simulink model "sm_motor_grader"  (R2026a)
settings: Solver=daessc  StopTime=stopTime  FixedStep=0.01  AbsTol=1e-3
PostLoadFcn:
  | warning off SimulinkBlock:Foundation:RuntimeAccessInvalidSource
InitFcn:
  | sm_motor_grader_config_initLinkBarHole([bdroot '/Motor Grader'],motGradParams)
StartFcn:
  | tic
StopFcn:
  | Elapsed_Sim_Time = toc;
undefined symbols (not defined in the file): Art, Center, Circle, FL, FR, Grid, LiftL, LiftR, LnL, LnR, Loads, motGradParams, Pin, RFL, RFR, RRL, RRR, Side, StrL, StrR, Tilt, Wheels
libraries: sm_motor_grader_lib x23, sm_lib x11, nesl_utility x10, fl_lib x2, sm_vehicle_utilities_lib x2
(part 2 of 2)

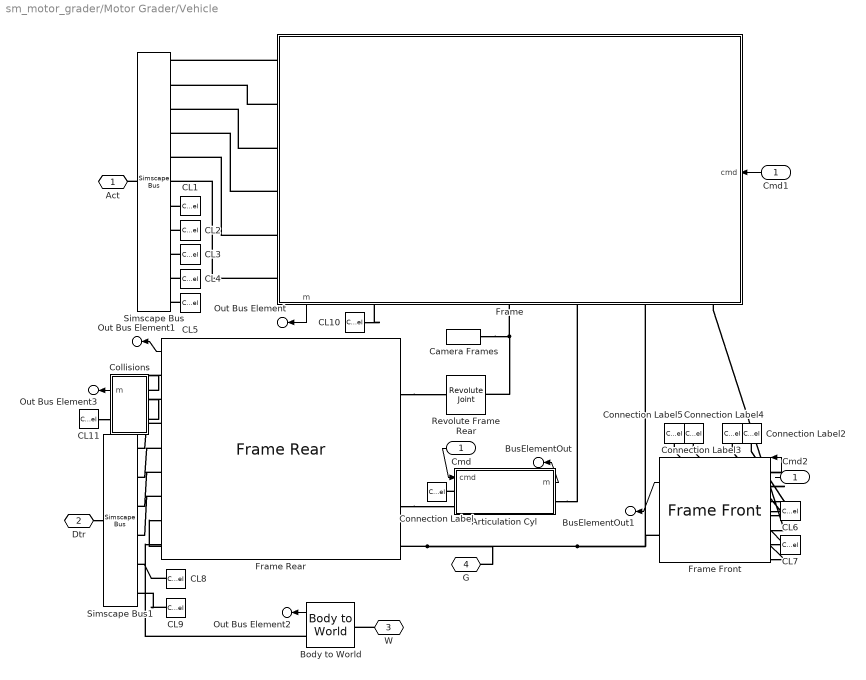
== system sm_motor_grader/Motor Grader/Vehicle ==
  Cmd : Inport
  Articulation Cyl : Subsystem  mask{popup_actuator_model=Position}
      mask prompts: popup_actuator_model "Actuation Mode"
      mask init:
      | bh = gcb;
      | if(strcmp(get_param(bh,'popup_actuator_model'),'Shaft'))
      |     set_param([bh '/Actuator'],'LabelModeActiveChoice','Shaft')
      | else
      |     set_param([bh '/Actuator'],'LabelModeActiveChoice','Position')
      | end
      settings: AttributesFormatString=%<popup_actuator_model>
      mask TypeOptions popup_actuator_model: Position | Shaft
      mask Display:
      | bh = gcb;
      | if(strcmp(get_param(bh,'popup_actuator_model'),'Position'))
      |     image('sm_motor_grader_actuator_intfPosition_IMAGE.png')
      | else
      |     image('sm_motor_grader_actuator_intfShaft_IMAGE.png')
      | end
      | %image('sm_motor_grader_articCylRod_IMAGE.png')
  Body to World : sm_vehicle_utilities_lib/Body to World  Init=Init.Vehicle  SpecifyPosTarget=on
  CL1 : ConnectionLabel  Label=Art
  CL10 : ConnectionLabel  Label=Gbl
  CL11 : ConnectionLabel  Label=Gbl
  CL2 : ConnectionLabel  Label=StrL
  CL3 : ConnectionLabel  Label=LnL
  CL4 : ConnectionLabel  Label=LnR
  CL5 : ConnectionLabel  Label=StrR
  CL6 : ConnectionLabel  Label=FL
  CL7 : ConnectionLabel  Label=FR
  CL8 : ConnectionLabel  Label=FL
  CL9 : ConnectionLabel  Label=FR
  Camera Frames : sm_vehicle_utilities_lib/Camera Frames  Camera=Camera  popup_dolly_camera=Off
  Cmd1 : InportShadow
  Cmd2 : InportShadow
  Collisions : Subsystem
  Connection Label : ConnectionLabel  Label=Art
  Connection Label2 : ConnectionLabel  Label=StrR
  Connection Label3 : ConnectionLabel  Label=LnR
  Connection Label4 : ConnectionLabel  Label=LnL
  Connection Label5 : ConnectionLabel  Label=StrL
  Frame : Subsystem  mask{popup_actuator_model=Position, popup_actuator_model_lift=Position, popup_initial_hole=Center, popup_blade_ground_contact=Loads}
      mask prompts: popup_actuator_model "Actuation Mode"; popup_actuator_model_lift "Actuation Mode Lift"; popup_initial_hole "Link Bar Initial Hole"; popup_blade_ground_contact "Blade Ground Contact"
      mask init:
      | bh = gcb;
      | 
      | modestr = get_param(bh,'popup_actuator_model');
      | set_param([bh '/Blade'],'popup_actuator_model',modestr)
      | set_param([bh '/Drawbar'],'popup_actuator_model',modestr)
      | set_param([bh '/LiftAssembly'],'popup_actuator_model',modestr)
      | 
      | liftmodestr = get_param(bh,'popup_actuator_model_lift');
      | set_param([bh '/LiftAssembly'],'popup_actuator_model_lift',liftmodestr)
      settings: PortSchema="{\"entries\":[{\"content\":{\"sides\":[{\"content\":{},\"type\":\"ConnectorPlacement.EquallySpacedRectSide\",\"uuid\":\"956ff1aa-cf24-496e-9779-d98cb55dab7e\"},{\"content\":{\"connectorIds\":[\"Out1\",\"RConn1\",\"RConn2\",\"RConn3\",\"RConn4\",\"RConn5\",\"RConn6\"],\"side\":\"RIGHT\"},\"type\":\"ConnectorPlacement.EquallySpacedRectSide\",\"uuid\":\"9c9b4268-8eee-41b9-b50a-4033054aa2f0\"},{\"content\":{\"connectorIds\":[\"LConn1\",\"LConn2\",\"LConn3\",\"LConn4\",\"LConn5\",\"LConn6\"],\"side\":\"TOP\"},\"type\":\"ConnectorPlacement.EquallySpacedRectSide\",\"uuid\":\"ed4b7b74-ed0a-49ca-b139-bba335fa3413\"},{\"content\":{\"connectorIds\":[\"In1\"],\"side\":\"BOTTOM\"},\"type\":\"ConnectorPlacement.EquallySpacedRectSide\",\"uuid\":\"cd037d6e-8d6c-4a0e-a629-b4586db15f4a\"}]},\"type\":\"ConnectorPlacement.EquallySpacedConnector\",\"uuid\":\"3490148e-7dca-48b7-9597-0781f6c140f1\"}],\"packageUris\":[\"http://schema.mathworks.com/mf0/Connector/R2020b\"],\"version\":\"1.0\"}"
      mask TypeOptions popup_actuator_model: Position | Shaft
      mask TypeOptions popup_actuator_model_lift: Position | Shaft
      mask TypeOptions popup_initial_hole: LiftAssembly/popup_initial_hole
      mask TypeOptions popup_blade_ground_contact: Blade/popup_blade_ground_contact
      mask Display: image('sm_motor_grader_frameCabBlade_IMAGE.png')
  Frame Front : sm_motor_grader_lib/Frame Front  popup_actuator_model=Position  popup_ground_contact=Magic Formula
  Frame Rear : sm_motor_grader_lib/Frame Rear  popup_ground_contact=Magic Formula
  Revolute Frame Rear : sm_lib/Joints/Revolute Joint  JointMode=Normal  CompositeWrenchDir=FollowerOnBase  CompositeWrenchFrame=BaseFrame  SenseConstraintForce=off  SenseConstraintTorque=off  SenseTotalForce=off  SenseTotalTorque=off  PositionTargetSpecify=on  PositionTargetPriority=Low  PositionTargetValue=0  PositionTargetValueUnits=deg  VelocityTargetSpecify=off  VelocityTargetPriority=High  VelocityTargetValue=0  VelocityTargetValueUnits=deg/s  EquilibriumPosition=0  EquilibriumPositionUnits=deg  SpringStiffness=0  SpringStiffnessUnits=N*m/deg  DampingCoefficient=0  DampingCoefficientUnits=N*m/(deg/s)  LowerLimitSpecify=off  LowerLimitBound=-90  LowerLimitBoundUnits=deg  LowerLimitStiffness=1e4  LowerLimitStiffnessUnits=N*m/deg  LowerLimitDamping=10  LowerLimitDampingUnits=N*m/(deg/s)  LowerLimitTransitionRegionWidth=0.1  LowerLimitTransitionRegionWidthUnits=deg  UpperLimitSpecify=off  UpperLimitBound=90  UpperLimitBoundUnits=deg  UpperLimitStiffness=1e4  UpperLimitStiffnessUnits=N*m/deg  UpperLimitDamping=10  UpperLimitDampingUnits=N*m/(deg/s)  UpperLimitTransitionRegionWidth=0.1  UpperLimitTransitionRegionWidthUnits=deg  TorqueActuationMode=NoTorque  MotionActuationMode=ComputedMotion  SensePosition=off  SenseVelocity=off  SenseAcceleration=off  SenseTorqueForce=off  SenseLowerLimitTorqueForce=off  SenseUpperLimitTorqueForce=off
  Simscape Bus : SimscapeBus  HierarchyStrings=Tilt;Side;Circle;LiftL;LiftR;Pin;Art;StrL;LnL;LnR;StrR
  Simscape Bus1 : SimscapeBus  HierarchyStrings=RFL;RFR;RRL;RRR;FL;FR
  Act : PMIOPort  Side=Left
  Dtr : PMIOPort  Port=2  Side=Left
  W : PMIOPort  Port=3  Side=Right
  G : PMIOPort  Port=4  Side=Right
  Out Bus Element : Outport  PortName=m  Element=Frame
  BusElementOut : Outport  PortName=m  Element=Artic
  BusElementOut1 : Outport  PortName=m  Element=FrameF
  Out Bus Element1 : Outport  PortName=m  Element=FrameR
  Out Bus Element2 : Outport  PortName=m  Element=World
  Out Bus Element3 : Outport  PortName=m  Element=Sep
  wires:
  Cmd/1 -> Articulation Cyl/1(cmd)
  Frame/1(m) -> Out Bus Element/1
  Articulation Cyl/1(m) -> BusElementOut/1
  Frame Front/1 -> BusElementOut1/1
  Frame Rear/1 -> Out Bus Element1/1
  Cmd1/1 -> Frame/1(cmd)
  Cmd2/1 -> Frame Front/1
  Body to World/1 -> Out Bus Element2/1
  Collisions/1(m) -> Out Bus Element3/1
  connections:
  Frame Front/RConn1 -- Frame/RConn5 -- G/RConn1 -- Frame Rear/RConn7
  Camera Frames/RConn1 -- Revolute Frame Rear/RConn1 -- Frame/RConn3
  Body to World/RConn1 -- Frame Rear/RConn8
  Frame Rear/LConn2 -- Articulation Cyl/LConn2
  Frame Rear/LConn1 -- Revolute Frame Rear/LConn1
  Articulation Cyl/RConn1 -- Frame/RConn4
  W/RConn1 -- Body to World/LConn1
  Articulation Cyl/LConn1 -- Connection Label/LConn1
  Simscape Bus/RConn1 -- Act/RConn1
  Frame/LConn1 -- Simscape Bus/LConn1
  Frame/LConn2 -- Simscape Bus/LConn2
  Frame Front/LConn5 -- Frame/RConn6
  Frame/LConn3 -- Simscape Bus/LConn3
  Frame/LConn4 -- Simscape Bus/LConn4
  Frame/LConn5 -- Simscape Bus/LConn5
  Frame Front/LConn3 -- Connection Label2/LConn1
  Frame Front/LConn4 -- Connection Label3/LConn1
  Frame Front/LConn6 -- Connection Label4/LConn1
  Frame Front/LConn7 -- Connection Label5/LConn1
  CL1/LConn1 -- Simscape Bus/LConn7
  CL3/LConn1 -- Simscape Bus/LConn9
  CL2/LConn1 -- Simscape Bus/LConn8
  CL4/LConn1 -- Simscape Bus/LConn10
  CL5/LConn1 -- Simscape Bus/LConn11
  Frame Rear/RConn3 -- Simscape Bus1/LConn1
  Frame Rear/RConn4 -- Simscape Bus1/LConn2
  Frame Rear/RConn5 -- Simscape Bus1/LConn3
  Frame Rear/RConn6 -- Simscape Bus1/LConn4
  Dtr/RConn1 -- Simscape Bus1/RConn1
  Frame Front/LConn1 -- CL6/LConn1
  Frame Front/LConn2 -- CL7/LConn1
  CL8/LConn1 -- Simscape Bus1/LConn5
  CL9/LConn1 -- Simscape Bus1/LConn6
  Frame/LConn6 -- Simscape Bus/LConn6
  Frame Rear/RConn1 -- Collisions/LConn1
  Frame Rear/RConn2 -- Collisions/LConn2
  CL10/LConn1 -- Frame/RConn1
  CL11/LConn1 -- Collisions/RConn1

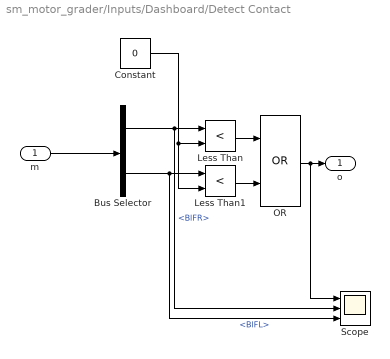
== system sm_motor_grader/Inputs/Dashboard/Detect Contact ==
  m : Inport
  Bus Selector : BusSelector  OutputSignals=Vehicle.Sep.BlFR,Vehicle.Sep.BlFL
  Constant : Constant  Value=0
  Less Than : RelationalOperator  Operator=<  OutDataTypeStr=boolean  RndMeth=Simplest  InputSameDT=off
  Less Than1 : RelationalOperator  Operator=<  OutDataTypeStr=boolean  RndMeth=Simplest  InputSameDT=off
  OR : Logic  Operator=OR  AllPortsSameDT=off  OutDataTypeStr=fixdt(1,16)
  Scope : Scope  NumInputPorts=3
      settings: ActiveDisplayYMinimum=-0.20528  ActiveDisplayYMaximum=1.8475
  o : Outport
  wires:
  m/1 -> Bus Selector/1
  Bus Selector/1 -> Scope/2, Less Than/1  "<BlFR>"
  Bus Selector/2 -> Scope/3, Less Than1/1  "<BlFL>"
  Constant/1 -> Less Than1/2, Less Than/2
  Less Than1/1 -> OR/2
  Less Than/1 -> OR/1
  OR/1 -> Scope/1, o/1

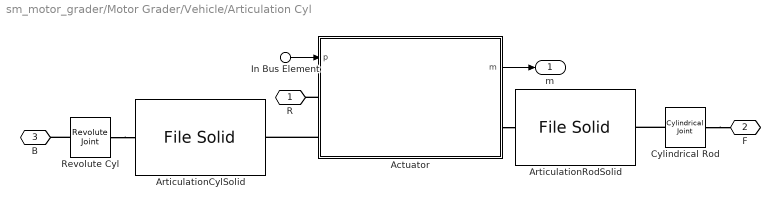
== system sm_motor_grader/Motor Grader/Vehicle/Articulation Cyl ==
  In Bus Element : Inport  PortName=cmd  Element=pArtic
  Actuator : Subsystem  Variant=on  VariantControlMode=label  VariantControl=Position  LabelModeActiveChoice=Position
  ArticulationCylSolid : sm_lib/Body Elements/File Solid  ExtGeomFileName=ArticulationCylinder.step  UnitType=FromFile  ExtGeomFileUnits=m  StepReaderType=HEX  ExportConvexHullGeometry=off  InertiaType=CalculateFromGeometry  BasedOnType=Mass  Density=1000  DensityUnits=kg/m^3  Mass=motGradParams.articulation.cyl.mass  MassUnits=kg  CenterOfMass=[0 0 0]  CenterOfMassUnits=m  MomentsOfInertia=[1 1 1]  MomentsOfInertiaUnits=kg*m^2  ProductsOfInertia=[0 0 0]  ProductsOfInertiaUnits=kg*m^2  GraphicType=FromGeometry  MarkerShape=Sphere  MarkerSize=10  GraphicVisPropType=SimpleVisualProperties  GraphicDiffuseColor=mtrgrd.clr.artic_cyl  GraphicOpacity=0.5  GraphicSpecularColor=[0.5 0.5 0.5 1.0]  GraphicAmbientColor=[0.15 0.15 0.15 1.0]  GraphicEmissiveColor=[0.0 0.0 0.0 1.0]  GraphicShininess=75  DoExposeReferenceFrame=off  SerializedFrames=<Frames><Frame><Id>Frame1</Id><Value><Name>MainFrameRev</Name><Origin><Source>GeometricFeature</Source><FeatureName>circular curve 11</FeatureName></Origin><PrimaryAxis><DefinedDirection>-Z</DefinedDirection><Source>GeometricFeature</Source><SourceDirection>+Z</SourceDirection><FeatureName>segment 13</FeatureName></PrimaryAxis><SecondaryAxis><DefinedDirection>+X</DefinedDirection><Source>ReferenceFrame</Source><SourceDirection>+X</SourceDirection><FeatureName></FeatureName></SecondaryAxis></Value></Frame><Frame><Id>Frame2</Id><Value><Name>ArticulationCyl</Name><Origin><Source>GeometricFeature</Source><FeatureName>circular curve 5</FeatureName></Origin><PrimaryAxis><DefinedDirection>-Z</DefinedDirection><Source>GeometricFeature</Source><SourceDirection>+Z</SourceDirection><FeatureName>segment 7</FeatureName></PrimaryAxis><SecondaryAxis><DefinedDirection>+X</DefinedDirection><Source>ReferenceFrame</Source><SourceDirection>+X</SourceDirection><FeatureName></FeatureName></SecondaryAxis></Value></Frame></Frames>
  ArticulationRodSolid : sm_lib/Body Elements/File Solid  ExtGeomFileName=ArticulationPiston.step  UnitType=FromFile  ExtGeomFileUnits=m  StepReaderType=HEX  ExportConvexHullGeometry=off  InertiaType=CalculateFromGeometry  BasedOnType=Mass  Density=1000  DensityUnits=kg/m^3  Mass=motGradParams.articulation.rod.mass  MassUnits=kg  CenterOfMass=[0 0 0]  CenterOfMassUnits=m  MomentsOfInertia=[1 1 1]  MomentsOfInertiaUnits=kg*m^2  ProductsOfInertia=[0 0 0]  ProductsOfInertiaUnits=kg*m^2  GraphicType=FromGeometry  MarkerShape=Sphere  MarkerSize=10  GraphicVisPropType=SimpleVisualProperties  GraphicDiffuseColor=mtrgrd.clr.artic_rod  GraphicOpacity=1  GraphicSpecularColor=[0.5 0.5 0.5 1.0]  GraphicAmbientColor=[0.15 0.15 0.15 1.0]  GraphicEmissiveColor=[0.0 0.0 0.0 1.0]  GraphicShininess=75  DoExposeReferenceFrame=off  SerializedFrames=<Frames><Frame><Id>Frame1</Id><Value><Name>RearFrame</Name><Origin><Source>GeometricFeature</Source><FeatureName>circular curve 4</FeatureName></Origin><PrimaryAxis><DefinedDirection>+Z</DefinedDirection><Source>ReferenceFrame</Source><SourceDirection>+Z</SourceDirection><FeatureName></FeatureName></PrimaryAxis><SecondaryAxis><DefinedDirection>+X</DefinedDirection><Source>ReferenceFrame</Source><SourceDirection>+X</SourceDirection><FeatureName></FeatureName></SecondaryAxis></Value></Frame><Frame><Id>Frame2</Id><Value><Name>ArticulationCyl</Name><Origin><Source>GeometricFeature</Source><FeatureName>planar surface 1</FeatureName></Origin><PrimaryAxis><DefinedDirection>-Z</DefinedDirection><Source>GeometricFeature</Source><SourceDirection>+Z</SourceDirection><FeatureName>segment 10</FeatureName></PrimaryAxis><SecondaryAxis><DefinedDirection>+X</DefinedDirection><Source>ReferenceFrame</Source><SourceDirection>+X</SourceDirection><FeatureName></FeatureName></SecondaryAxis></Value></Frame></Frames>
  Cylindrical Rod : sm_lib/Joints/Cylindrical Joint  JointMode=Normal  CompositeWrenchDir=FollowerOnBase  CompositeWrenchFrame=BaseFrame  SenseConstraintForce=off  SenseConstraintTorque=off  SenseTotalForce=off  SenseTotalTorque=off  RzPositionTargetSpecify=off  RzPositionTargetPriority=High  RzPositionTargetValue=0  RzPositionTargetValueUnits=deg  RzVelocityTargetSpecify=off  RzVelocityTargetPriority=High  RzVelocityTargetValue=0  RzVelocityTargetValueUnits=deg/s  RzEquilibriumPosition=0  RzEquilibriumPositionUnits=deg  RzSpringStiffness=0  RzSpringStiffnessUnits=N*m/deg  RzDampingCoefficient=0  RzDampingCoefficientUnits=N*m/(deg/s)  RzLowerLimitSpecify=off  RzLowerLimitBound=-90  RzLowerLimitBoundUnits=deg  RzLowerLimitStiffness=1e4  RzLowerLimitStiffnessUnits=N*m/deg  RzLowerLimitDamping=10  RzLowerLimitDampingUnits=N*m/(deg/s)  RzLowerLimitTransitionRegionWidth=0.1  RzLowerLimitTransitionRegionWidthUnits=deg  RzUpperLimitSpecify=off  RzUpperLimitBound=90  RzUpperLimitBoundUnits=deg  RzUpperLimitStiffness=1e4  RzUpperLimitStiffnessUnits=N*m/deg  RzUpperLimitDamping=10  RzUpperLimitDampingUnits=N*m/(deg/s)  RzUpperLimitTransitionRegionWidth=0.1  RzUpperLimitTransitionRegionWidthUnits=deg  RzTorqueActuationMode=NoTorque  RzMotionActuationMode=ComputedMotion  RzSensePosition=off  RzSenseVelocity=off  RzSenseAcceleration=off  RzSenseTorqueForce=off  RzSenseLowerLimitTorqueForce=off  RzSenseUpperLimitTorqueForce=off  PzPositionTargetSpecify=off  PzPositionTargetPriority=High  PzPositionTargetValue=0  PzPositionTargetValueUnits=m  PzVelocityTargetSpecify=off  PzVelocityTargetPriority=High  PzVelocityTargetValue=0  PzVelocityTargetValueUnits=m/s  PzEquilibriumPosition=0  PzEquilibriumPositionUnits=m  PzSpringStiffness=0  PzSpringStiffnessUnits=N/m  PzDampingCoefficient=0  PzDampingCoefficientUnits=N/(m/s)  PzLowerLimitSpecify=off  PzLowerLimitBound=-1  PzLowerLimitBoundUnits=m  PzLowerLimitStiffness=1e6  PzLowerLimitStiffnessUnits=N/m  PzLowerLimitDamping=1e3  PzLowerLimitDampingUnits=N/(m/s)  PzLowerLimitTransitionRegionWidth=1e-4  PzLowerLimitTransitionRegionWidthUnits=m  PzUpperLimitSpecify=off  PzUpperLimitBound=1  PzUpperLimitBoundUnits=m  PzUpperLimitStiffness=1e6  PzUpperLimitStiffnessUnits=N/m  PzUpperLimitDamping=1e3  PzUpperLimitDampingUnits=N/(m/s)  PzUpperLimitTransitionRegionWidth=1e-4  PzUpperLimitTransitionRegionWidthUnits=m  PzTorqueActuationMode=NoTorque  PzMotionActuationMode=ComputedMotion  PzSensePosition=off  PzSenseVelocity=off  PzSenseAcceleration=off  PzSenseTorqueForce=off  PzSenseLowerLimitTorqueForce=off  PzSenseUpperLimitTorqueForce=off
  Revolute Cyl : sm_lib/Joints/Revolute Joint  JointMode=Normal  CompositeWrenchDir=FollowerOnBase  CompositeWrenchFrame=BaseFrame  SenseConstraintForce=off  SenseConstraintTorque=off  SenseTotalForce=off  SenseTotalTorque=off  PositionTargetSpecify=off  PositionTargetPriority=High  PositionTargetValue=0  PositionTargetValueUnits=deg  VelocityTargetSpecify=off  VelocityTargetPriority=High  VelocityTargetValue=0  VelocityTargetValueUnits=deg/s  EquilibriumPosition=0  EquilibriumPositionUnits=deg  SpringStiffness=0  SpringStiffnessUnits=N*m/deg  DampingCoefficient=0  DampingCoefficientUnits=N*m/(deg/s)  LowerLimitSpecify=off  LowerLimitBound=-90  LowerLimitBoundUnits=deg  LowerLimitStiffness=1e4  LowerLimitStiffnessUnits=N*m/deg  LowerLimitDamping=10  LowerLimitDampingUnits=N*m/(deg/s)  LowerLimitTransitionRegionWidth=0.1  LowerLimitTransitionRegionWidthUnits=deg  UpperLimitSpecify=off  UpperLimitBound=90  UpperLimitBoundUnits=deg  UpperLimitStiffness=1e4  UpperLimitStiffnessUnits=N*m/deg  UpperLimitDamping=10  UpperLimitDampingUnits=N*m/(deg/s)  UpperLimitTransitionRegionWidth=0.1  UpperLimitTransitionRegionWidthUnits=deg  TorqueActuationMode=NoTorque  MotionActuationMode=ComputedMotion  SensePosition=off  SenseVelocity=off  SenseAcceleration=off  SenseTorqueForce=off  SenseLowerLimitTorqueForce=off  SenseUpperLimitTorqueForce=off
  R : PMIOPort  Side=Left
  F : PMIOPort  Port=2  Side=Left
  B : PMIOPort  Port=3  Side=Right
  m : Outport
  wires:
  In Bus Element/1 -> Actuator/1(p)
  Actuator/1(m) -> m/1
  connections:
  Revolute Cyl/RConn1 -- ArticulationCylSolid/LConn1
  Revolute Cyl/LConn1 -- B/RConn1
  Cylindrical Rod/LConn1 -- F/RConn1
  Cylindrical Rod/RConn1 -- ArticulationRodSolid/LConn1
  Actuator/LConn1 -- R/RConn1
  Actuator/LConn2 -- ArticulationCylSolid/RConn1
  Actuator/RConn1 -- ArticulationRodSolid/RConn1

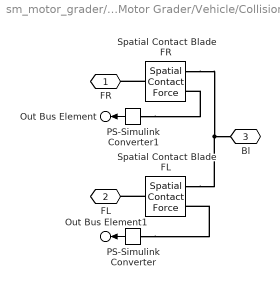
== system sm_motor_grader/Motor Grader/Vehicle/Collisions ==
  PS-Simulink Converter : nesl_utility/PS-Simulink Converter  PhysicalDomain=network_engine_domain  SubClassName=ps_output  LeftPortType=input  RightPortType=output  PseudoPeriodic=off  Frequencies=[]  VectorFormat=inherit  Unit=inherit  AffineConversion=off
  PS-Simulink Converter1 : nesl_utility/PS-Simulink Converter  PhysicalDomain=network_engine_domain  SubClassName=ps_output  LeftPortType=input  RightPortType=output  PseudoPeriodic=off  Frequencies=[]  VectorFormat=inherit  Unit=inherit  AffineConversion=off
  Spatial Contact Blade FL : sm_lib/Forces and Torques/Spatial Contact Force  SenseSeparationDistance=on  NormalForceType=SmoothSpringDamper  NormalStiffness=0  NormalStiffnessUnits=N/m  NormalDamping=0  NormalDampingUnits=N/(m/s)  NormalTransitionRegionWidth=10  NormalTransitionRegionWidthUnits=m  FrictionType=SmoothStickSlip  CoefficientOfStaticFriction=0  CoefficientOfDynamicFriction=0  FrictionalCriticalVelocity=10  FrictionalCriticalVelocityUnits=m/s  SenseContactSignal=off  SensePenetrationDepth=off  SenseNormalVelocity=off  SenseTangentialVelocity=off  SensingForceTorqueDirection=BaseOnFollower  SensingForceTorqueResolutionFrame=ContactFrame  SenseNormalForce=off  SenseNormalForceMagnitude=off  SenseNormalTorque=off  SenseFrictionalForce=off  SenseFrictionalForceMagnitude=off  SenseFrictionalTorque=off  SenseTotalForce=off  SenseTotalTorque=off  SenseContactBaseRotation=off  SenseContactBaseTranslation=off  SenseContactFollowerRotation=off  SenseContactFollowerTranslation=off  ZeroCrossDetectContactStartAndEnd=off
  Spatial Contact Blade FR : sm_lib/Forces and Torques/Spatial Contact Force  SenseSeparationDistance=on  NormalForceType=SmoothSpringDamper  NormalStiffness=0  NormalStiffnessUnits=N/m  NormalDamping=0  NormalDampingUnits=N/(m/s)  NormalTransitionRegionWidth=10  NormalTransitionRegionWidthUnits=m  FrictionType=SmoothStickSlip  CoefficientOfStaticFriction=0  CoefficientOfDynamicFriction=0  FrictionalCriticalVelocity=10  FrictionalCriticalVelocityUnits=m/s  SenseContactSignal=off  SensePenetrationDepth=off  SenseNormalVelocity=off  SenseTangentialVelocity=off  SensingForceTorqueDirection=BaseOnFollower  SensingForceTorqueResolutionFrame=ContactFrame  SenseNormalForce=off  SenseNormalForceMagnitude=off  SenseNormalTorque=off  SenseFrictionalForce=off  SenseFrictionalForceMagnitude=off  SenseFrictionalTorque=off  SenseTotalForce=off  SenseTotalTorque=off  SenseContactBaseRotation=off  SenseContactBaseTranslation=off  SenseContactFollowerRotation=off  SenseContactFollowerTranslation=off  ZeroCrossDetectContactStartAndEnd=off
  FR : PMIOPort  Side=Left
  FL : PMIOPort  Port=2  Side=Left
  Bl : PMIOPort  Port=3  Side=Right
  Out Bus Element : Outport  PortName=m  Element=BlFR
  Out Bus Element1 : Outport  PortName=m  Element=BlFL
  wires:
  PS-Simulink Converter1/1 -> Out Bus Element/1
  PS-Simulink Converter/1 -> Out Bus Element1/1
  connections:
  Spatial Contact Blade FR/LConn1 -- FR/RConn1
  Spatial Contact Blade FR/RConn1 -- Spatial Contact Blade FL/RConn1 -- Bl/RConn1
  Spatial Contact Blade FL/LConn1 -- FL/RConn1
  PS-Simulink Converter/LConn1 -- Spatial Contact Blade FL/RConn2
  PS-Simulink Converter1/LConn1 -- Spatial Contact Blade FR/RConn2

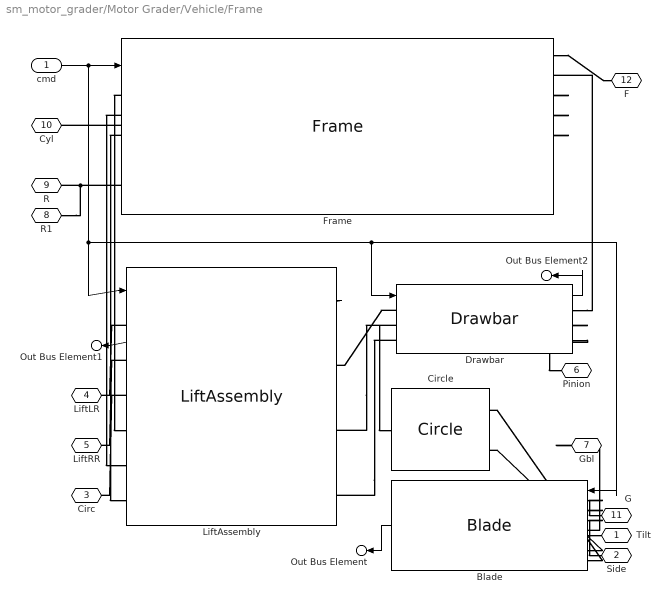
== system sm_motor_grader/Motor Grader/Vehicle/Frame ==
  cmd : Inport
  Blade : sm_motor_grader_lib/Blade  popup_actuator_model=Position  popup_blade_ground_contact=Loads
      settings: AttributesFormatString=%<popup_actuator_model>
  Circle : sm_motor_grader_lib/Circle
  Drawbar : sm_motor_grader_lib/Drawbar  popup_actuator_model=Position
      settings: AttributesFormatString=%<popup_actuator_model>
  Frame : sm_motor_grader_lib/Frame
  LiftAssembly : sm_motor_grader_lib/LiftAssembly  popup_actuator_model=Position  popup_actuator_model_lift=Position  popup_initial_hole=Center
      settings: AttributesFormatString=|
      | Circle: %<popup_actuator_model>
      | Lift: %<popup_actuator_model_lift>
  Tilt : PMIOPort  Side=Left
  Side : PMIOPort  Port=2  Side=Left
  Circ : PMIOPort  Port=3  Side=Left
  LiftLR : PMIOPort  Port=4  Side=Left
  LiftRR : PMIOPort  Port=5  Side=Left
  Pinion : PMIOPort  Port=6  Side=Left
  Gbl : PMIOPort  Port=7  Side=Right
  R1 : PMIOPort  Port=8  Side=Right
  R : PMIOPort  Port=9  Side=Right
  Cyl : PMIOPort  Port=10  Side=Right
  G : PMIOPort  Port=11  Side=Right
  F : PMIOPort  Port=12  Side=Right
  Out Bus Element : Outport  PortName=m  Element=Blade
  Out Bus Element1 : Outport  PortName=m  Element=Lift
  Out Bus Element2 : Outport  PortName=m  Element=Drawbar
  wires:
  cmd/1 -> Frame/1, LiftAssembly/1, Drawbar/1, Blade/1
  Blade/1 -> Out Bus Element/1
  LiftAssembly/1 -> Out Bus Element1/1
  Drawbar/1 -> Out Bus Element2/1
  connections:
  Blade/LConn1 -- G/RConn1
  Drawbar/RConn2 -- Circle/LConn1
  Drawbar/LConn3 -- LiftAssembly/RConn3
  Blade/LConn6 -- Circle/RConn2
  Frame/RConn3 -- LiftAssembly/LConn4
  Drawbar/LConn1 -- LiftAssembly/RConn1
  Drawbar/LConn2 -- LiftAssembly/RConn2
  Drawbar/RConn1 -- Frame/RConn2
  Frame/RConn5 -- LiftAssembly/LConn6
  Blade/LConn7 -- Circle/RConn1
  Frame/RConn4 -- LiftAssembly/LConn5
  Frame/LConn1 -- Cyl/RConn1
  Frame/RConn1 -- F/RConn1
  R1/RConn1 -- Frame/LConn2 -- R/RConn1
  Blade/LConn2 -- Tilt/RConn1
  Blade/LConn3 -- Side/RConn1
  LiftAssembly/LConn3 -- Circ/RConn1
  LiftAssembly/LConn1 -- LiftLR/RConn1
  LiftAssembly/LConn2 -- LiftRR/RConn1
  Drawbar/RConn3 -- Pinion/RConn1
  Gbl/RConn1 -- Blade/LConn4

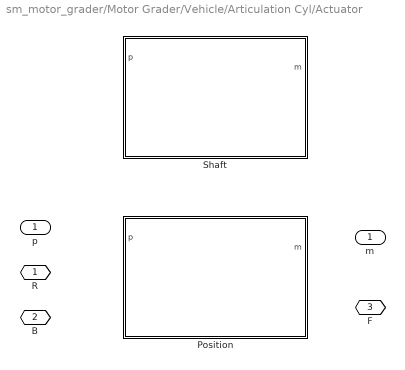
== system sm_motor_grader/Motor Grader/Vehicle/Articulation Cyl/Actuator ==
  p : Inport
  Position : Subsystem  VariantControl=Position
      mask Display: image('sm_motor_grader_cyljoint_Position_IMAGE.png')
  Shaft : Subsystem  VariantControl=Shaft
      mask Display: image('sm_motor_grader_cyljoint_Shaft_IMAGE.png')
  R : PMIOPort  Side=Left
  B : PMIOPort  Port=2  Side=Left
  F : PMIOPort  Port=3  Side=Right
  m : Outport

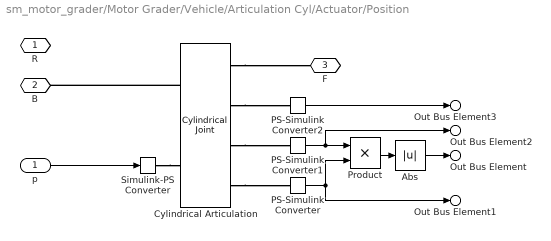
== system sm_motor_grader/Motor Grader/Vehicle/Articulation Cyl/Actuator/Position ==
  p : Inport
  Abs : Abs  ZeroCross=off  SaturateOnIntegerOverflow=off
  Cylindrical Articulation : sm_lib/Joints/Cylindrical Joint  JointMode=Normal  CompositeWrenchDir=FollowerOnBase  CompositeWrenchFrame=BaseFrame  SenseConstraintForce=off  SenseConstraintTorque=off  SenseTotalForce=off  SenseTotalTorque=off  RzPositionTargetSpecify=off  RzPositionTargetPriority=High  RzPositionTargetValue=0  RzPositionTargetValueUnits=deg  RzVelocityTargetSpecify=off  RzVelocityTargetPriority=High  RzVelocityTargetValue=0  RzVelocityTargetValueUnits=deg/s  RzEquilibriumPosition=0  RzEquilibriumPositionUnits=deg  RzSpringStiffness=0  RzSpringStiffnessUnits=N*m/deg  RzDampingCoefficient=0  RzDampingCoefficientUnits=N*m/(deg/s)  RzLowerLimitSpecify=off  RzLowerLimitBound=-90  RzLowerLimitBoundUnits=deg  RzLowerLimitStiffness=1e4  RzLowerLimitStiffnessUnits=N*m/deg  RzLowerLimitDamping=10  RzLowerLimitDampingUnits=N*m/(deg/s)  RzLowerLimitTransitionRegionWidth=0.1  RzLowerLimitTransitionRegionWidthUnits=deg  RzUpperLimitSpecify=off  RzUpperLimitBound=90  RzUpperLimitBoundUnits=deg  RzUpperLimitStiffness=1e4  RzUpperLimitStiffnessUnits=N*m/deg  RzUpperLimitDamping=10  RzUpperLimitDampingUnits=N*m/(deg/s)  RzUpperLimitTransitionRegionWidth=0.1  RzUpperLimitTransitionRegionWidthUnits=deg  RzTorqueActuationMode=NoTorque  RzMotionActuationMode=ComputedMotion  RzSensePosition=off  RzSenseVelocity=off  RzSenseAcceleration=off  RzSenseTorqueForce=off  RzSenseLowerLimitTorqueForce=off  RzSenseUpperLimitTorqueForce=off  PzPositionTargetSpecify=on  PzPositionTargetPriority=High  PzPositionTargetValue=motGradParams.articulation.initPos  PzPositionTargetValueUnits=m  PzVelocityTargetSpecify=off  PzVelocityTargetPriority=High  PzVelocityTargetValue=0  PzVelocityTargetValueUnits=m/s  PzEquilibriumPosition=0  PzEquilibriumPositionUnits=m  PzSpringStiffness=0  PzSpringStiffnessUnits=N/m  PzDampingCoefficient=0  PzDampingCoefficientUnits=N/(m/s)  PzLowerLimitSpecify=on  PzLowerLimitBound=motGradParams.articulation.lowerBound  PzLowerLimitBoundUnits=m  PzLowerLimitStiffness=1e6  PzLowerLimitStiffnessUnits=N/m  PzLowerLimitDamping=1e3  PzLowerLimitDampingUnits=N/(m/s)  PzLowerLimitTransitionRegionWidth=1e-4  PzLowerLimitTransitionRegionWidthUnits=m  PzUpperLimitSpecify=on  PzUpperLimitBound=motGradParams.articulation.upperBound  PzUpperLimitBoundUnits=m  PzUpperLimitStiffness=1e6  PzUpperLimitStiffnessUnits=N/m  PzUpperLimitDamping=1e3  PzUpperLimitDampingUnits=N/(m/s)  PzUpperLimitTransitionRegionWidth=1e-4  PzUpperLimitTransitionRegionWidthUnits=m  PzTorqueActuationMode=ComputedTorque  PzMotionActuationMode=InputMotion  PzSensePosition=on  PzSenseVelocity=on  PzSenseAcceleration=off  PzSenseTorqueForce=on  PzSenseLowerLimitTorqueForce=off  PzSenseUpperLimitTorqueForce=off
  PS-Simulink Converter : nesl_utility/PS-Simulink Converter  PhysicalDomain=network_engine_domain  SubClassName=ps_output  LeftPortType=input  RightPortType=output  PseudoPeriodic=off  Frequencies=[]  VectorFormat=inherit  Unit=inherit  AffineConversion=off
  PS-Simulink Converter1 : nesl_utility/PS-Simulink Converter  PhysicalDomain=network_engine_domain  SubClassName=ps_output  LeftPortType=input  RightPortType=output  PseudoPeriodic=off  Frequencies=[]  VectorFormat=inherit  Unit=inherit  AffineConversion=off
  PS-Simulink Converter2 : nesl_utility/PS-Simulink Converter  PhysicalDomain=network_engine_domain  SubClassName=ps_output  LeftPortType=input  RightPortType=output  PseudoPeriodic=off  Frequencies=[]  VectorFormat=inherit  Unit=inherit  AffineConversion=off
  Product : Product
  Simulink-PS Converter : nesl_utility/Simulink-PS Converter  PhysicalDomain=network_engine_domain  SubClassName=ps_input  LeftPortType=input  RightPortType=output  PseudoPeriodic=off  Frequencies=[]  NoiseDistribution=none  NoiseParameters=[]  Unit=1  AffineConversion=off  FilteringAndDerivatives=filter  SimscapeFilterOrder=2  InputFilterTimeConstant=0.001  UdotUserProvided=0
  R : PMIOPort  Side=Left
  B : PMIOPort  Port=2  Side=Left
  F : PMIOPort  Port=3  Side=Right
  Out Bus Element : Outport  PortName=m  Element=power
  Out Bus Element1 : Outport  PortName=m  Element=force
  Out Bus Element2 : Outport  PortName=m  Element=v
  Out Bus Element3 : Outport  PortName=m  Element=p
  wires:
  p/1 -> Simulink-PS Converter/1
  Product/1 -> Abs/1
  PS-Simulink Converter1/1 -> Out Bus Element2/1, Product/1
  PS-Simulink Converter/1 -> Out Bus Element1/1, Product/2
  Abs/1 -> Out Bus Element/1
  PS-Simulink Converter2/1 -> Out Bus Element3/1
  connections:
  Cylindrical Articulation/RConn1 -- F/RConn1
  Simulink-PS Converter/RConn1 -- Cylindrical Articulation/LConn2
  Cylindrical Articulation/LConn1 -- B/RConn1
  Cylindrical Articulation/RConn2 -- PS-Simulink Converter2/LConn1
  Cylindrical Articulation/RConn3 -- PS-Simulink Converter1/LConn1
  Cylindrical Articulation/RConn4 -- PS-Simulink Converter/LConn1

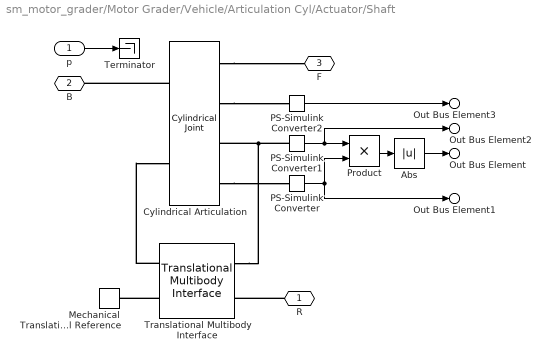
== system sm_motor_grader/Motor Grader/Vehicle/Articulation Cyl/Actuator/Shaft ==
  p : Inport
  Abs : Abs  ZeroCross=off  SaturateOnIntegerOverflow=off
  Cylindrical Articulation : sm_lib/Joints/Cylindrical Joint  JointMode=Normal  CompositeWrenchDir=FollowerOnBase  CompositeWrenchFrame=BaseFrame  SenseConstraintForce=off  SenseConstraintTorque=off  SenseTotalForce=off  SenseTotalTorque=off  RzPositionTargetSpecify=off  RzPositionTargetPriority=High  RzPositionTargetValue=0  RzPositionTargetValueUnits=deg  RzVelocityTargetSpecify=off  RzVelocityTargetPriority=High  RzVelocityTargetValue=0  RzVelocityTargetValueUnits=deg/s  RzEquilibriumPosition=0  RzEquilibriumPositionUnits=deg  RzSpringStiffness=0  RzSpringStiffnessUnits=N*m/deg  RzDampingCoefficient=0  RzDampingCoefficientUnits=N*m/(deg/s)  RzLowerLimitSpecify=off  RzLowerLimitBound=-90  RzLowerLimitBoundUnits=deg  RzLowerLimitStiffness=1e4  RzLowerLimitStiffnessUnits=N*m/deg  RzLowerLimitDamping=10  RzLowerLimitDampingUnits=N*m/(deg/s)  RzLowerLimitTransitionRegionWidth=0.1  RzLowerLimitTransitionRegionWidthUnits=deg  RzUpperLimitSpecify=off  RzUpperLimitBound=90  RzUpperLimitBoundUnits=deg  RzUpperLimitStiffness=1e4  RzUpperLimitStiffnessUnits=N*m/deg  RzUpperLimitDamping=10  RzUpperLimitDampingUnits=N*m/(deg/s)  RzUpperLimitTransitionRegionWidth=0.1  RzUpperLimitTransitionRegionWidthUnits=deg  RzTorqueActuationMode=NoTorque  RzMotionActuationMode=ComputedMotion  RzSensePosition=off  RzSenseVelocity=off  RzSenseAcceleration=off  RzSenseTorqueForce=off  RzSenseLowerLimitTorqueForce=off  RzSenseUpperLimitTorqueForce=off  PzPositionTargetSpecify=on  PzPositionTargetPriority=High  PzPositionTargetValue=motGradParams.articulation.initPos  PzPositionTargetValueUnits=m  PzVelocityTargetSpecify=off  PzVelocityTargetPriority=High  PzVelocityTargetValue=0  PzVelocityTargetValueUnits=m/s  PzEquilibriumPosition=0  PzEquilibriumPositionUnits=m  PzSpringStiffness=0  PzSpringStiffnessUnits=N/m  PzDampingCoefficient=0  PzDampingCoefficientUnits=N/(m/s)  PzLowerLimitSpecify=on  PzLowerLimitBound=motGradParams.articulation.lowerBound  PzLowerLimitBoundUnits=m  PzLowerLimitStiffness=1e6  PzLowerLimitStiffnessUnits=N/m  PzLowerLimitDamping=1e3  PzLowerLimitDampingUnits=N/(m/s)  PzLowerLimitTransitionRegionWidth=1e-4  PzLowerLimitTransitionRegionWidthUnits=m  PzUpperLimitSpecify=on  PzUpperLimitBound=motGradParams.articulation.upperBound  PzUpperLimitBoundUnits=m  PzUpperLimitStiffness=1e6  PzUpperLimitStiffnessUnits=N/m  PzUpperLimitDamping=1e3  PzUpperLimitDampingUnits=N/(m/s)  PzUpperLimitTransitionRegionWidth=1e-4  PzUpperLimitTransitionRegionWidthUnits=m  PzTorqueActuationMode=InputTorque  PzMotionActuationMode=ComputedMotion  PzSensePosition=on  PzSenseVelocity=on  PzSenseAcceleration=off  PzSenseTorqueForce=on  PzSenseLowerLimitTorqueForce=off  PzSenseUpperLimitTorqueForce=off
  Mechanical Translational Reference : fl_lib/Mechanical/Translational Elements/Mechanical Translational Reference
  PS-Simulink Converter : nesl_utility/PS-Simulink Converter  PhysicalDomain=network_engine_domain  SubClassName=ps_output  LeftPortType=input  RightPortType=output  PseudoPeriodic=off  Frequencies=[]  VectorFormat=inherit  Unit=inherit  AffineConversion=off
  PS-Simulink Converter1 : nesl_utility/PS-Simulink Converter  PhysicalDomain=network_engine_domain  SubClassName=ps_output  LeftPortType=input  RightPortType=output  PseudoPeriodic=off  Frequencies=[]  VectorFormat=inherit  Unit=inherit  AffineConversion=off
  PS-Simulink Converter2 : nesl_utility/PS-Simulink Converter  PhysicalDomain=network_engine_domain  SubClassName=ps_output  LeftPortType=input  RightPortType=output  PseudoPeriodic=off  Frequencies=[]  VectorFormat=inherit  Unit=inherit  AffineConversion=off
  Product : Product
  Terminator : Terminator
  Translational Multibody Interface : fl_lib/Mechanical/Multibody Interfaces/Translational Multibody Interface
  R : PMIOPort  Side=Left
  B : PMIOPort  Port=2  Side=Left
  F : PMIOPort  Port=3  Side=Right
  Out Bus Element : Outport  PortName=m  Element=power
  Out Bus Element1 : Outport  PortName=m  Element=force
  Out Bus Element2 : Outport  PortName=m  Element=v
  Out Bus Element3 : Outport  PortName=m  Element=p
  wires:
  p/1 -> Terminator/1
  Product/1 -> Abs/1
  PS-Simulink Converter/1 -> Out Bus Element1/1, Product/2
  Abs/1 -> Out Bus Element/1
  PS-Simulink Converter2/1 -> Out Bus Element3/1
  PS-Simulink Converter1/1 -> Out Bus Element2/1, Product/1
  connections:
  Cylindrical Articulation/LConn1 -- B/RConn1
  Cylindrical Articulation/RConn1 -- F/RConn1
  Translational Multibody Interface/RConn1 -- Cylindrical Articulation/RConn3 -- PS-Simulink Converter1/LConn1
  Translational Multibody Interface/LConn1 -- Cylindrical Articulation/LConn2
  Translational Multibody Interface/LConn2 -- Mechanical Translational Reference/LConn1
  R/RConn1 -- Translational Multibody Interface/RConn2
  Cylindrical Articulation/RConn2 -- PS-Simulink Converter2/LConn1
  Cylindrical Articulation/RConn4 -- PS-Simulink Converter/LConn1
